simulink model "SMC_network"  (R2021a)
settings: Solver=VariableStepAuto  StartTime=0.0  StopTime=5  RelTol=1e-3
values from neighbouring files (symbols this model uses):
  C = 1e-12    [SMCCodes.m]
  eta_d = 1e27    (= 1e+27)    [SMCCodes.m]
  eta_ds = 1e5    (= 100000)    [SMCCodes.m]
  eta_q = 1e27    (= 1e+27)    [SMCCodes.m]
  eta_qs = 1e5    (= 100000)    [SMCCodes.m]
  g = -10e14    (= -1e+15)    [SMCCodes.m]
  gs = -1/Lt    (= -99.6909580301)    [SMCCodes.m]
  L = 100e-3    (= 0.1)    [SMCCodes.m]
  lambda = 1e10    (= 10000000000)    [SMCCodes.m]
  Lf = 10e-3    (= 0.01)    [SMCCodes.m]
  Lg = 0    [SMCCodes.m]
  Ll = 31e-6    (= 3.1e-05)    [SMCCodes.m]
  phi = 0.01    [SMCCodes.m]
  R = 4.33    [SMCCodes.m]
  Rf = 40e-3    (= 0.04)    [SMCCodes.m]
  RL = 0.1    [SMCCodes.m]
  Ts = 0.50e-5    (= 5e-06)    [SMCCodes.m]
undefined symbols (not defined in the file or in its folder): Ion, Lithium, sigbuilder_block
libraries: spsMeanLib x47, spsSeriesRLCBranchLib x23, simulink x22, spsFirstOrderFilterLib x10, spsIGBTDiodeLib x8, pid_lib x8, spsPWMGeneratorDCDCLib x8, spsabctodq0Lib x7, spsThreePhaseVIMeasurementLib x6, spsCurrentMeasurementLib x4, spsDiodeLib x4, spsIGBTLib x4
(part 3 of 3)

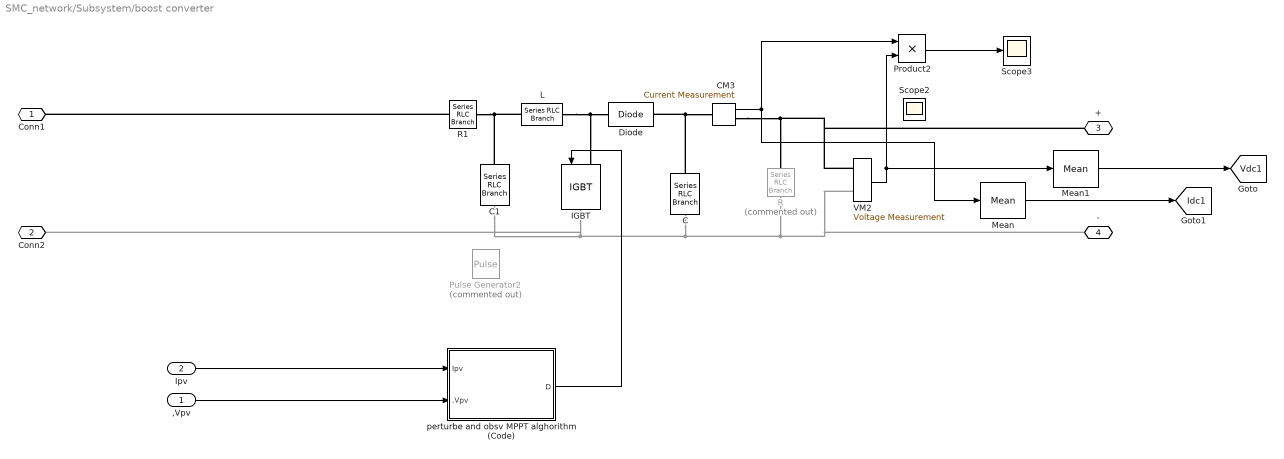
== system SMC_network/Subsystem/boost converter ==
  ,Vpv : Inport
  "Ipv " : Inport  Port=2
  C : spsSeriesRLCBranchLib/Series RLC Branch  LConnTagsString=__new0  RConnTagsString=__new0  BranchType=C  Resistance=0.01  Inductance=1.0  SetiL0=off  InitialCurrent=0  Capacitance=500e-6  Setx0=off  InitialVoltage=200  Measurements=None
  C1 : spsSeriesRLCBranchLib/Series RLC Branch  LConnTagsString=__new0  RConnTagsString=__new0  BranchType=C  Resistance=0.01  Inductance=1.0  SetiL0=off  InitialCurrent=0  Capacitance=1000e-6  Setx0=off  InitialVoltage=34.5  Measurements=None
  CM3 : spsCurrentMeasurementLib/Current Measurement  Tag=PoWeRsYsTeMmEaSuReMeNt  PhasorSimulation=off  OutputType=Magnitude  PSBequivalent=0
      settings: AttributesFormatString=\n
  Diode : spsDiodeLib/Diode  Ron=0.001  Lon=0  Vf=0.8  IC=0  UseSnubber=0  Rs=500  Cs=250e-9  Measurements=off
      settings: AttributesFormatString=\n
  IGBT : spsIGBTLib/IGBT  Ron=0.001  Lon=0  Vf=1  Tf=1e-6  Tt=2e-6  IC=0  Rs=1e5  Cs=inf  Measurements=off
  L : spsSeriesRLCBranchLib/Series RLC Branch  LConnTagsString=__new0  RConnTagsString=__new0  BranchType=L  Resistance=1.0  Inductance=168e-6  SetiL0=off  InitialCurrent=0  Capacitance=1.0  Setx0=off  InitialVoltage=0  Measurements=None
  Mean : spsMeanLib/Mean  Freq=60  Vinit=0  Ts=0
  Mean1 : spsMeanLib/Mean  Freq=60  Vinit=0  Ts=0
  Product2 : Product  RndMeth=Zero
  Pulse Generator2 : DiscretePulseGenerator  Commented=on  PulseType=Time based  Amplitude=2  Period=1/1000  PulseWidth=35
  R : spsSeriesRLCBranchLib/Series RLC Branch  Commented=on  LConnTagsString=__new0  RConnTagsString=__new0  BranchType=R  Resistance=10  Inductance=1.0  SetiL0=off  InitialCurrent=0  Capacitance=1.0  Setx0=off  InitialVoltage=0  Measurements=None
  R1 : spsSeriesRLCBranchLib/Series RLC Branch  LConnTagsString=__new0  RConnTagsString=__new0  BranchType=R  Resistance=1  Inductance=1.0  SetiL0=off  InitialCurrent=0  Capacitance=1.0  Setx0=off  InitialVoltage=0  Measurements=None
  Scope2 : Scope
  Scope3 : Scope
  VM2 : spsVoltageMeasurementLib/Voltage Measurement  Tag=PoWeRsYsTeMmEaSuReMeNt  PhasorSimulation=off  OutputType=Magnitude  PSBequivalent=0
  perturbe and obsv MPPT alghorithm (Code) : Subsystem
  Conn1 : PMIOPort  Side=Left
  Conn2 : PMIOPort  Port=2  Side=Left
  + : PMIOPort  Port=3  Side=Right
  - : PMIOPort  Port=4  Side=Right
  tag scope: Idc1=global, Vdc1=global
  wires:
  CM3/1 -> Mean/1, Product2/1
  VM2/1 -> Mean1/1, Product2/2
  perturbe and obsv MPPT alghorithm (Code)/1(D) -> IGBT/1
  Product2/1 -> Scope3/1
  "Ipv "/1 -> perturbe and obsv MPPT alghorithm (Code)/1("Ipv ")
  ,Vpv/1 -> perturbe and obsv MPPT alghorithm (Code)/2(,Vpv)
  Mean/1 -> [Idc1]
  Mean1/1 -> [Vdc1]
  connections:
  L/LConn1 -- R1/RConn1 -- C1/LConn1
  R/RConn1 -- -/RConn1 -- VM2/LConn2 -- C1/RConn1 -- Conn2/RConn1 -- IGBT/RConn1 -- C/RConn1
  L/RConn1 -- Diode/LConn1 -- IGBT/LConn1
  C/LConn1 -- CM3/LConn1 -- Diode/RConn1
  CM3/RConn1 -- R/LConn1 -- VM2/LConn1 -- +/RConn1
  R1/LConn1 -- Conn1/RConn1

== system SMC_network/Subsystem/boost converter1 ==
  ,Vpv : Inport
  "Ipv " : Inport  Port=2
  C : spsSeriesRLCBranchLib/Series RLC Branch  LConnTagsString=__new0  RConnTagsString=__new0  BranchType=C  Resistance=0.01  Inductance=1.0  SetiL0=off  InitialCurrent=0  Capacitance=500e-6  Setx0=off  InitialVoltage=200  Measurements=None
  C1 : spsSeriesRLCBranchLib/Series RLC Branch  LConnTagsString=__new0  RConnTagsString=__new0  BranchType=C  Resistance=0.01  Inductance=1.0  SetiL0=off  InitialCurrent=0  Capacitance=1000e-6  Setx0=off  InitialVoltage=34.5  Measurements=None
  CM3 : spsCurrentMeasurementLib/Current Measurement  Tag=PoWeRsYsTeMmEaSuReMeNt  PhasorSimulation=off  OutputType=Magnitude  PSBequivalent=0
      settings: AttributesFormatString=\n
  Diode : spsDiodeLib/Diode  Ron=0.00001  Lon=0  Vf=0.8  IC=0  UseSnubber=0  Rs=500  Cs=250e-9  Measurements=off
      settings: AttributesFormatString=\n
  IGBT : spsIGBTLib/IGBT  Ron=0.00001  Lon=0  Vf=1  Tf=1e-6  Tt=2e-6  IC=0  Rs=1e5  Cs=inf  Measurements=off
  L : spsSeriesRLCBranchLib/Series RLC Branch  LConnTagsString=__new0  RConnTagsString=__new0  BranchType=L  Resistance=1.0  Inductance=168e-6  SetiL0=off  InitialCurrent=0  Capacitance=1.0  Setx0=off  InitialVoltage=0  Measurements=None
  Mean : spsMeanLib/Mean  Freq=60  Vinit=0  Ts=0
  Mean1 : spsMeanLib/Mean  Freq=60  Vinit=0  Ts=0
  Product2 : Product  RndMeth=Zero
  Pulse Generator2 : DiscretePulseGenerator  Commented=on  PulseType=Time based  Amplitude=2  Period=1/1000  PulseWidth=35
  R : spsSeriesRLCBranchLib/Series RLC Branch  Commented=on  LConnTagsString=__new0  RConnTagsString=__new0  BranchType=R  Resistance=10  Inductance=1.0  SetiL0=off  InitialCurrent=0  Capacitance=1.0  Setx0=off  InitialVoltage=0  Measurements=None
  R1 : spsSeriesRLCBranchLib/Series RLC Branch  LConnTagsString=__new0  RConnTagsString=__new0  BranchType=R  Resistance=1  Inductance=1.0  SetiL0=off  InitialCurrent=0  Capacitance=1.0  Setx0=off  InitialVoltage=0  Measurements=None
  Scope2 : Scope
  Scope3 : Scope
  VM2 : spsVoltageMeasurementLib/Voltage Measurement  Tag=PoWeRsYsTeMmEaSuReMeNt  PhasorSimulation=off  OutputType=Magnitude  PSBequivalent=0
  perturbe and obsv MPPT alghorithm (Code) : Subsystem
  Conn1 : PMIOPort  Side=Left
  Conn2 : PMIOPort  Port=2  Side=Left
  + : PMIOPort  Port=3  Side=Right
  - : PMIOPort  Port=4  Side=Right
  tag scope: Idc2=global, Vdc2=global
  wires:
  ,Vpv/1 -> perturbe and obsv MPPT alghorithm (Code)/2(,Vpv)
  "Ipv "/1 -> perturbe and obsv MPPT alghorithm (Code)/1("Ipv ")
  Product2/1 -> Scope3/1
  perturbe and obsv MPPT alghorithm (Code)/1(D) -> IGBT/1
  VM2/1 -> Product2/2, Mean1/1
  CM3/1 -> Mean/1, Scope2/1, Product2/1
  Mean1/1 -> [Vdc2]
  Mean/1 -> [Idc2]
  connections:
  R1/LConn1 -- Conn1/RConn1
  +/RConn1 -- VM2/LConn1 -- R/LConn1 -- CM3/RConn1
  Diode/RConn1 -- CM3/LConn1 -- C/LConn1
  IGBT/LConn1 -- Diode/LConn1 -- L/RConn1
  C/RConn1 -- IGBT/RConn1 -- Conn2/RConn1 -- C1/RConn1 -- VM2/LConn2 -- -/RConn1 -- R/RConn1
  C1/LConn1 -- R1/RConn1 -- L/LConn1

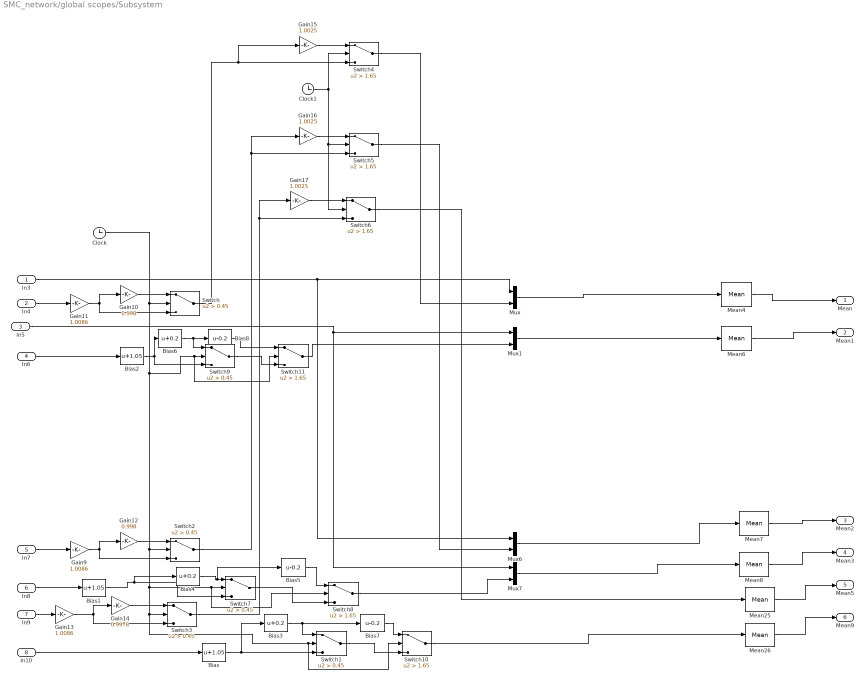
== system SMC_network/global scopes/Subsystem ==
  In3 : Inport
  In4 : Inport  Port=2
  In5 : Inport  Port=3
  In6 : Inport  Port=4
  In7 : Inport  Port=5
  In8 : Inport  Port=6
  In9 : Inport  Port=7
  In10 : Inport  Port=8
  Bias : Bias  Bias=1.05  SaturateOnIntegerOverflow=on
  Bias1 : Bias  Bias=1.05  SaturateOnIntegerOverflow=on
  Bias2 : Bias  Bias=1.05  SaturateOnIntegerOverflow=on
  Bias3 : Bias  Bias=0.2  SaturateOnIntegerOverflow=on
  Bias4 : Bias  Bias=0.2  SaturateOnIntegerOverflow=on
  Bias5 : Bias  Bias=-0.2  SaturateOnIntegerOverflow=on
  Bias6 : Bias  Bias=0.2  SaturateOnIntegerOverflow=on
  Bias7 : Bias  Bias=-0.2  SaturateOnIntegerOverflow=on
  Bias8 : Bias  Bias=-0.2  SaturateOnIntegerOverflow=on
  Clock : Clock
  Clock1 : Clock
  Gain10 : Gain  Gain=0.998
  Gain11 : Gain  Gain=1.0086
  Gain12 : Gain  Gain=0.998
  Gain13 : Gain  Gain=1.0086
  Gain14 : Gain  Gain=0.9978
  Gain15 : Gain  Gain=1.0025
  Gain16 : Gain  Gain=1.0025
  Gain17 : Gain  Gain=1.0025
  Gain9 : Gain  Gain=1.0086
  Mean{4,6..8,25..26} (6 alike) : spsMeanLib/Mean  Freq=50  Vinit=0  Ts=0
  Mux{,1,6..7} (4 alike) : Mux  Inputs=2
  Switch{,1..3,7,9} (6 alike) : Switch  Criteria=u2 > Threshold  Threshold=0.45
  Switch{4..6,8,10..11} (6 alike) : Switch  Criteria=u2 > Threshold  Threshold=1.65
  Mean : Outport
  Mean1 : Outport  Port=2
  Mean2 : Outport  Port=3
  Mean3 : Outport  Port=4
  Mean5 : Outport  Port=5
  Mean9 : Outport  Port=6
  wires:
  In3/1 -> Mux6/1, Mux/1
  In4/1 -> Gain11/1
  Clock/1 -> Switch11/2, Switch9/2, Switch2/2, Switch10/2, Switch1/2, Switch3/2, Switch8/2, Switch7/2, Switch/2
  Switch/1 -> Gain15/1, Switch4/3
  Switch2/1 -> Switch5/3, Gain16/1
  Switch3/1 -> Gain17/1, Switch6/3
  Mean4/1 -> Mean/1
  Mean8/1 -> Mean3/1
  Gain17/1 -> Switch6/1
  Gain14/1 -> Switch3/1
  Gain13/1 -> Switch3/3, Gain14/1
  Clock1/1 -> Switch4/2, Switch6/2, Switch5/2
  Gain16/1 -> Switch5/1
  In5/1 -> Mux1/1, Mux7/1
  Switch6/1 -> Mean25/1
  Mux/1 -> Mean4/1
  Mux6/1 -> Mean7/1
  Mux7/1 -> Mean8/1
  Mux1/1 -> Mean6/1
  Gain11/1 -> Switch/3, Gain10/1
  Gain15/1 -> Switch4/1
  Gain9/1 -> Gain12/1, Switch2/3
  Switch4/1 -> Mux/2
  In9/1 -> Gain13/1
  In10/1 -> Bias/1
  Mean25/1 -> Mean5/1
  Gain10/1 -> Switch/1
  Gain12/1 -> Switch2/1
  Mean26/1 -> Mean9/1
  Switch5/1 -> Mux6/2
  Mean7/1 -> Mean2/1
  Mean6/1 -> Mean1/1
  In7/1 -> Gain9/1
  In8/1 -> Bias1/1
  In6/1 -> Bias2/1
  Bias/1 -> Bias3/1, Switch1/3
  Bias3/1 -> Bias7/1, Switch1/1
  Bias1/1 -> Bias4/1, Switch7/3
  Bias4/1 -> Bias5/1, Switch7/1
  Bias5/1 -> Switch8/1
  Switch7/1 -> Switch8/3
  Bias2/1 -> Bias6/1, Switch9/3
  Bias6/1 -> Bias8/1, Switch9/1
  Switch1/1 -> Switch10/3
  Bias7/1 -> Switch10/1
  Switch10/1 -> Mean26/1
  Switch8/1 -> Mux7/2
  Switch11/1 -> Mux1/2
  Switch9/1 -> Switch11/3
  Bias8/1 -> Switch11/1

== system SMC_network/global scopes/Subsystem1 ==
  In2 : Inport
  In1 : Inport  Port=2
  Bias : Bias  Bias=-1.7  SaturateOnIntegerOverflow=on
  Bias1 : Bias  Bias=-0.58  SaturateOnIntegerOverflow=on
  Bias2 : Bias  Bias=0.5  SaturateOnIntegerOverflow=on
  Bias3 : Bias  SaturateOnIntegerOverflow=on
  Bias4 : Bias  Bias=-0.15  SaturateOnIntegerOverflow=on
  Bias5 : Bias  Bias=-0.6  SaturateOnIntegerOverflow=on
  Bias6 : Bias  Bias=-0.1  SaturateOnIntegerOverflow=on
  Bias7 : Bias  Bias=+0.1  SaturateOnIntegerOverflow=on
  Bias9 : Bias  Bias=+0.18  SaturateOnIntegerOverflow=on
  Clock : Clock
  Switch : Switch  Criteria=u2 > Threshold  Threshold=1.03
  Switch1 : Switch  Criteria=u2 > Threshold  Threshold=2.03
  Switch2 : Switch  Criteria=u2 > Threshold  Threshold=1.03
  Switch3 : Switch  Criteria=u2 > Threshold  Threshold=4.03
  Switch4 : Switch  Criteria=u2 > Threshold  Threshold=2.03
  Switch5 : Switch  Criteria=u2 > Threshold  Threshold=3.03
  Switch7 : Switch  Criteria=u2 > Threshold  Threshold=4.03
  Out1 : Outport
  Out2 : Outport  Port=2
  wires:
  In2/1 -> Bias/1
  Clock/1 -> Switch4/2, Switch7/2, Switch5/2, Switch2/2, Switch1/2, Switch3/2, Switch/2
  Bias/1 -> Bias2/1, Switch/3
  Bias2/1 -> Bias3/1, Switch/1
  Bias3/1 -> Bias5/1, Switch1/1
  Switch/1 -> Switch1/3
  Bias1/1 -> Switch2/3, Bias4/1
  Bias4/1 -> Bias6/1, Switch2/1
  Bias5/1 -> Switch3/1
  Switch1/1 -> Switch3/3
  Switch2/1 -> Switch4/3
  Bias6/1 -> Bias7/1, Switch4/1
  Switch4/1 -> Switch5/3
  Bias7/1 -> Bias9/1, Switch5/1
  Switch5/1 -> Switch7/3
  Bias9/1 -> Switch7/1
  Switch7/1 -> Out2/1
  Switch3/1 -> Out1/1
  In1/1 -> Bias1/1

== system SMC_network/global scopes/Subsystem2 ==
  In1 : Inport
  In2 : Inport  Port=2
  Bias : Bias  Bias=-0.16  SaturateOnIntegerOverflow=on
  Bias1 : Bias  Bias=-0.04  SaturateOnIntegerOverflow=on
  Bias2 : Bias  Bias=-0.03  SaturateOnIntegerOverflow=on
  Bias3 : Bias  Bias=-0.01  SaturateOnIntegerOverflow=on
  Bias4 : Bias  Bias=+0.01
  Bias5 : Bias  Bias=-0.03  SaturateOnIntegerOverflow=on
  Bias6 : Bias  Bias=+0.03  SaturateOnIntegerOverflow=on
  Bias7 : Bias  Bias=+0.03  SaturateOnIntegerOverflow=on
  Clock : Clock
  Switch : Switch  Criteria=u2 > Threshold  Threshold=1
  Switch1 : Switch  Criteria=u2 > Threshold  Threshold=2.03
  Switch2 : Switch  Criteria=u2 > Threshold  Threshold=3.03
  Switch3 : Switch  Criteria=u2 > Threshold  Threshold=1
  Switch4 : Switch  Criteria=u2 > Threshold  Threshold=4.03
  Switch5 : Switch  Criteria=u2 > Threshold  Threshold=4.03
  Out1 : Outport
  Out2 : Outport  Port=2
  wires:
  In2/1 -> Bias1/1
  In1/1 -> Bias/1
  Clock/1 -> Switch4/2, Switch2/2, Switch1/2, Switch5/2, Switch3/2, Switch/2
  Bias1/1 -> Switch/3, Bias2/1
  Bias2/1 -> Bias3/1, Switch/1
  Switch/1 -> Switch1/3
  Bias3/1 -> Bias4/1, Switch1/1
  Switch1/1 -> Switch2/3
  Bias4/1 -> Bias6/1, Switch2/1
  Bias/1 -> Bias5/1, Switch3/3
  Bias5/1 -> Bias7/1, Switch3/1
  Switch2/1 -> Switch4/3
  Bias6/1 -> Switch4/1
  Switch4/1 -> Out2/1
  Switch3/1 -> Switch5/3
  Bias7/1 -> Switch5/1
  Switch5/1 -> Out1/1

== system SMC_network/refrences/Discrete Virtual PLL ==
  note: Pierre Giroux, Gilbert Sybille
      | Power System Simulation Laboratory
      | IREQ, Hydro-Quebc
  note: Discrete Virtual PLL
  Constant4 : Constant  Value=2*pi
  Deg->Rad : Gain  Gain=pi/180  SaturateOnIntegerOverflow=on  OutDataTypeStr=Inherit: Same as input  ParamDataTypeStr=Inherit: Same as input
  Freq1 : Constant  Value=Freq
  Freq2 : Constant  Value=2*pi
  Initial Vd_Vq1 : Constant  Value=Phase
  Math Function : Math  Operator=mod  SignedPower=on  SaturateOnIntegerOverflow=on
  Mux : Mux  Inputs=2
  Product : Product  Inputs=***  InputSameDT=on  SaturateOnIntegerOverflow=on  OutDataTypeStr=Inherit: Same as first input
  Sum : Sum  InputSameDT=on  SaturateOnIntegerOverflow=on  OutDataTypeStr=Inherit: Same as first input
  Trigonometric Function : Trigonometry
  Trigonometric Function1 : Trigonometry  Operator=cos
  t : DigitalClock  SampleTime=Ts
  Freq : Outport  VectorParamsAs1DForOutWhenUnconnected=off
  Sin_Cos : Outport  Port=2  VectorParamsAs1DForOutWhenUnconnected=off
  wt : Outport  Port=3  VectorParamsAs1DForOutWhenUnconnected=off
  wires:
  Sum/1 -> Math Function/1
  t/1 -> Product/2
  Freq2/1 -> Product/3
  Freq1/1 -> Product/1, Freq/1
  Deg->Rad/1 -> Sum/2
  Initial Vd_Vq1/1 -> Deg->Rad/1
  Product/1 -> Sum/1
  Constant4/1 -> Math Function/2
  Math Function/1 -> wt/1, Trigonometric Function1/1, Trigonometric Function/1
  Trigonometric Function/1 -> Mux/1
  Trigonometric Function1/1 -> Mux/2
  Mux/1 -> Sin_Cos/1

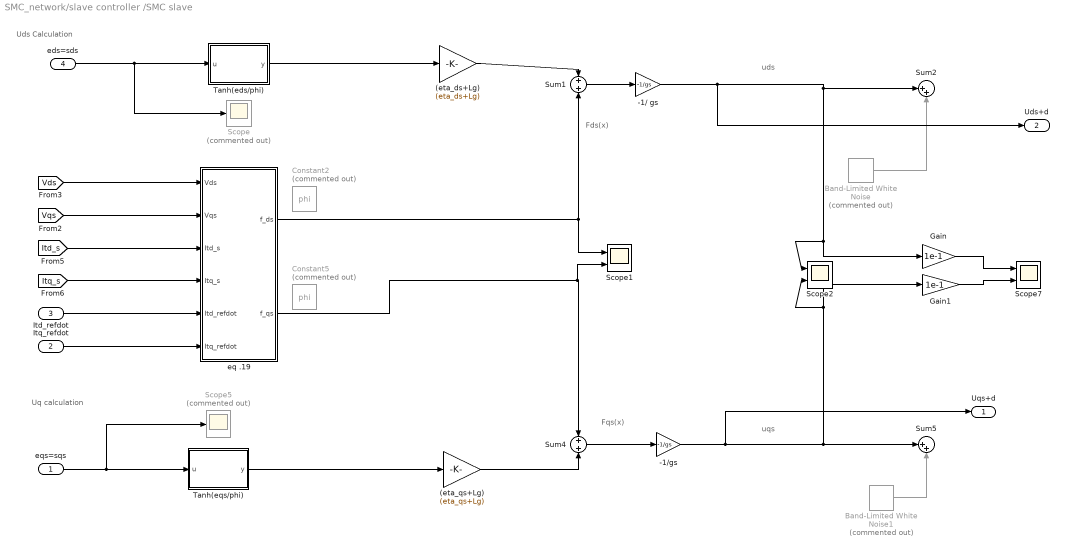
== system SMC_network/slave controller /SMC slave ==
  note: Uq calculation
  note: Uds Calculation
  note: uqs
  note: Fqs(x)
  note: Fds(x)
  note: uds
  eqs=sqs : Inport
  Itq_refdot : Inport  Port=2
  Itd_refdot : Inport  Port=3
  eds=sds : Inport  Port=4
  (eta_ds+Lg) : Gain  Gain=(eta_ds+Lg)
  (eta_qs+Lg) : Gain  Gain=(eta_qs+Lg)
  -1/ gs : Gain  Gain=-1/gs
  -1/gs : Gain  Gain=-1/gs
  Band-Limited White Noise : simulink/Sources/Band-Limited White Noise  Commented=on  Cov=[0.1]  Ts=0.002  seed=[21]
  Band-Limited White Noise1 : simulink/Sources/Band-Limited White Noise  Commented=on  Cov=[0.1]  Ts=0.002  seed=[23341]
  Constant2 : Constant  Commented=on  Value=phi
  Constant5 : Constant  Commented=on  Value=phi
  Gain : Gain  Gain=1e-1
  Gain1 : Gain  Gain=1e-1
  Scope : Scope  Commented=on
  Scope1 : Scope  NumInputPorts=2
  Scope2 : Scope  NumInputPorts=2
  Scope5 : Scope  Commented=on
  Scope7 : Scope  NumInputPorts=2
  Sum1 : Sum  Inputs=+|+
  Sum2 : Sum  Inputs=|++
  Sum4 : Sum
  Sum5 : Sum  Inputs=|++
  Tanh(eds/phi) : MATLAB Function  TreatAsAtomicUnit=on
  Tanh(eqs/phi) : MATLAB Function  TreatAsAtomicUnit=on
  eq .19 : MATLAB Function  TreatAsAtomicUnit=on
  Uqs+d : Outport
  Uds+d : Outport  Port=2
  wires:
  Tanh(eqs/phi)/1(y) -> (eta_qs+Lg)/1
  (eta_qs+Lg)/1 -> Sum4/2
  (eta_ds+Lg)/1 -> Sum1/1
  Tanh(eds/phi)/1(y) -> (eta_ds+Lg)/1
  Band-Limited White Noise1/1 -> Sum5/2
  -1/gs/1 -> Scope2/2, Gain1/1, Sum5/1, Uqs+d/1
  Sum4/1 -> -1/gs/1
  Band-Limited White Noise/1 -> Sum2/2
  -1/ gs/1 -> Uds+d/1, Gain/1, Scope2/1, Sum2/1
  Sum1/1 -> -1/ gs/1
  eds=sds/1 -> Scope/1, Tanh(eds/phi)/1(u)
  eqs=sqs/1 -> Scope5/1, Tanh(eqs/phi)/1(u)
  eq .19/1(f_ds) -> Scope1/1, Sum1/2
  eq .19/2(f_qs) -> Scope1/2, Sum4/1
  [Vds] -> eq .19/1(Vds)
  [Vqs] -> eq .19/2(Vqs)
  [Itd_s] -> eq .19/3(Itd_s)
  [Itq_s] -> eq .19/4(Itq_s)
  Itd_refdot/1 -> eq .19/5(Itd_refdot)
  Itq_refdot/1 -> eq .19/6(Itq_refdot)
  Gain/1 -> Scope7/1
  Gain1/1 -> Scope7/2

== system SMC_network/slave controller /calculation ==
  Itd_s_ref : Inport
  Itd_s : Inport  Port=2
  Discrete Derivative : simulink/Discrete/Discrete Derivative  Commented=on  gainval=1.0  ICPrevScaledInput=0.0  OutMin=[]  OutMax=[]  OutDataType=fixdt(1, 16)  OutScaling=2^-10  DoSatur=off
  First-Order Filter1 : spsFirstOrderFilterLib/First-Order Filter  FilterType=Lowpass  Tc=10e-3  Ts=0  Initialize=off  Vac_Init=[0, 0, 60]  Vdc_Init=0  PlotResponse=off  FreqRange="[0,  200,  1]"
  First-Order Filter2 : spsFirstOrderFilterLib/First-Order Filter  Commented=on  FilterType=Lowpass  Tc=20e-3  Ts=0  Initialize=off  Vac_Init=[0, 0, 60]  Vdc_Init=0  PlotResponse=off  FreqRange="[0,  200,  1]"
  Sum : Sum  Inputs=|+-
  XY Graph : simulink/Sinks/XY Graph  Commented=on  xmin=-2.5  xmax=2.5  ymin=-30  ymax=40  st=-1
  eds=sds : Outport
  tag scope: ed_s=global
  wires:
  Itd_s_ref/1 -> Sum/1
  Itd_s/1 -> Sum/2
  Sum/1 -> Discrete Derivative/1, XY Graph/1, [ed_s], eds=sds/1
  Discrete Derivative/1 -> First-Order Filter2/1
  First-Order Filter2/1 -> XY Graph/2

== system SMC_network/slave controller /calculation1 ==
  Itq_s_ref : Inport
  Itq_s : Inport  Port=2
  Discrete Derivative : simulink/Discrete/Discrete Derivative  Commented=on  gainval=1.0  ICPrevScaledInput=0.0  OutMin=[]  OutMax=[]  OutDataType=fixdt(1, 16)  OutScaling=2^-10  DoSatur=off
  First-Order Filter1 : spsFirstOrderFilterLib/First-Order Filter  Commented=on  FilterType=Lowpass  Tc=20e-3  Ts=0  Initialize=off  Vac_Init=[0, 0, 60]  Vdc_Init=0  PlotResponse=off  FreqRange="[0,  200,  1]"
  Sum : Sum  Inputs=|+-
  XY Graph : simulink/Sinks/XY Graph  Commented=on  xmin=-2.5  xmax=2.5  ymin=-20  ymax=30  st=-1
  eqs=sqs : Outport
  tag scope: eq_s=global
  wires:
  Itq_s_ref/1 -> Sum/1
  Itq_s/1 -> Sum/2
  Sum/1 -> XY Graph/1, [eq_s], eqs=sqs/1, Discrete Derivative/1
  Discrete Derivative/1 -> First-Order Filter1/1
  First-Order Filter1/1 -> XY Graph/2

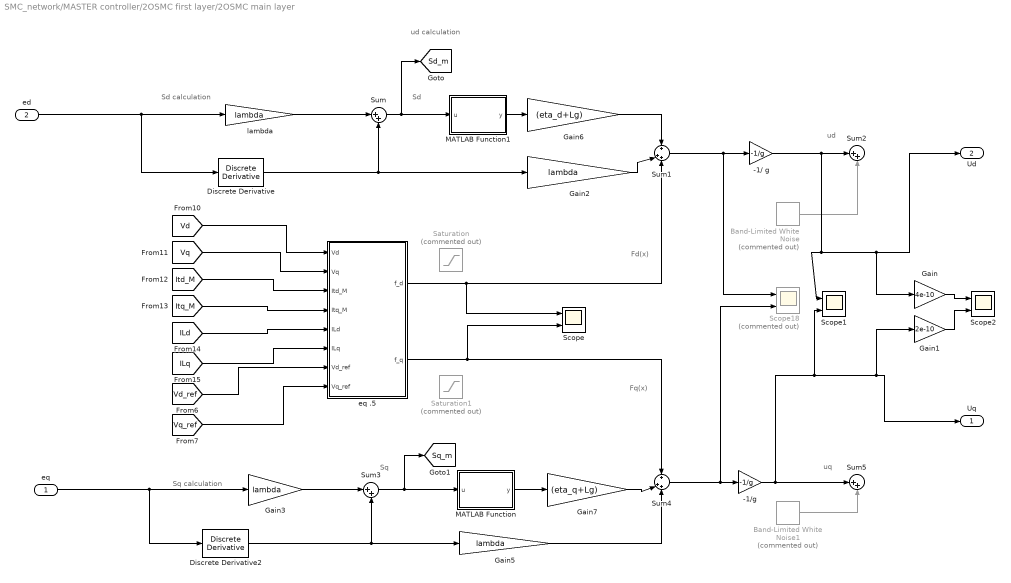
== system SMC_network/MASTER controller/2OSMC first layer/2OSMC main layer ==
  note: ud calculation
  note: ud
  note: Sq
  note: Fd(x)
  note: Sd
  note: Sd calculation
  note: Sq calculation
  note: Fq(x)
  note: uq
  eq : Inport
  ed : Inport  Port=2
  -1/ g : Gain  Gain=-1/g
  -1/g : Gain  Gain=-1/g
  Band-Limited White Noise : simulink/Sources/Band-Limited White Noise  Commented=on  Cov=[0.1]  Ts=0.002  seed=[21]
  Band-Limited White Noise1 : simulink/Sources/Band-Limited White Noise  Commented=on  Cov=[0.1]  Ts=0.002  seed=[23341]
  Discrete Derivative : simulink/Discrete/Discrete Derivative  gainval=1.0  ICPrevScaledInput=0.0  OutMin=[]  OutMax=[]  OutDataType=fixdt(1, 16)  OutScaling=2^-10  DoSatur=off
  Discrete Derivative2 : simulink/Discrete/Discrete Derivative  gainval=1.0  ICPrevScaledInput=0.0  OutMin=[]  OutMax=[]  OutDataType=fixdt(1, 16)  OutScaling=2^-10  DoSatur=off
  Gain : Gain  Gain=4e-10
  Gain1 : Gain  Gain=2e-10
  Gain2 : Gain  Gain=lambda
  Gain3 : Gain  Gain=lambda
  Gain5 : Gain  Gain=lambda
  Gain6 : Gain  Gain=(eta_d+Lg)
  Gain7 : Gain  Gain=(eta_q+Lg)
  MATLAB Function : MATLAB Function  TreatAsAtomicUnit=on
  MATLAB Function1 : MATLAB Function  TreatAsAtomicUnit=on
  Saturation : Saturate  Commented=on  UpperLimit=65e22  LowerLimit=0
  Saturation1 : Saturate  Commented=on  UpperLimit=110e12  LowerLimit=0
  Scope : Scope  NumInputPorts=2
  Scope1 : Scope  NumInputPorts=2
  Scope18 : Scope  Commented=on  NumInputPorts=2
  Scope2 : Scope  NumInputPorts=2
  Sum{,2..3,5} (4 alike) : Sum  Inputs=|++
  Sum1 : Sum  Inputs=+|++
  Sum4 : Sum  Inputs=+|++
  eq .5 : MATLAB Function  TreatAsAtomicUnit=on
  lambda : Gain  Gain=lambda
  Uq : Outport
  Ud : Outport  Port=2
  tag scope: Sd_m=global, Sq_m=global
  wires:
  ed/1 -> Discrete Derivative/1, lambda/1
  Gain2/1 -> Sum1/2
  Sum/1 -> [Sd_m], MATLAB Function1/1(u)
  Sum1/1 -> Scope18/1, -1/ g/1
  Band-Limited White Noise/1 -> Sum2/2
  Sum4/1 -> -1/g/1, Scope18/2
  Sum3/1 -> [Sq_m], MATLAB Function/1(u)
  Band-Limited White Noise1/1 -> Sum5/2
  MATLAB Function1/1(y) -> Gain6/1
  Gain6/1 -> Sum1/1
  Gain7/1 -> Sum4/2
  MATLAB Function/1(y) -> Gain7/1
  Gain5/1 -> Sum4/3
  eq/1 -> Discrete Derivative2/1, Gain3/1
  -1/g/1 -> Scope1/2, Gain1/1, Uq/1, Sum5/1
  -1/ g/1 -> Scope1/1, Ud/1, Gain/1, Sum2/1
  eq .5/2(f_q) -> Scope/2, Sum4/1
  eq .5/1(f_d) -> Sum1/3, Scope/1
  [Vd] -> eq .5/1(Vd)
  [Vq] -> eq .5/2(Vq)
  [Itd_M] -> eq .5/3(Itd_M)
  [Itq_M] -> eq .5/4(Itq_M)
  [ILd] -> eq .5/5(ILd)
  [ILq] -> eq .5/6(ILq)
  Discrete Derivative/1 -> Sum/2, Gain2/1
  lambda/1 -> Sum/1
  Gain3/1 -> Sum3/1
  Discrete Derivative2/1 -> Sum3/2, Gain5/1
  [Vd_ref] -> eq .5/7(Vd_ref)
  [Vq_ref] -> eq .5/8(Vq_ref)
  Gain1/1 -> Scope2/2
  Gain/1 -> Scope2/1

== system SMC_network/MASTER controller/2OSMC first layer/calculation ==
  Vd : Inport
  Vd_ref : Inport  Port=2
  Discrete Derivative : simulink/Discrete/Discrete Derivative  Commented=on  gainval=1.0  ICPrevScaledInput=0.0  OutMin=[]  OutMax=[]  OutDataType=fixdt(1, 16)  OutScaling=2^-10  DoSatur=off
  First-Order Filter : spsFirstOrderFilterLib/First-Order Filter  Commented=on  FilterType=Lowpass  Tc=20e-3  Ts=0  Initialize=off  Vac_Init=[0, 0, 60]  Vdc_Init=0  PlotResponse=off  FreqRange="[0,  200,  1]"
  Sum : Sum  Inputs=+-
  XY Graph : simulink/Sinks/XY Graph  Commented=on  xmin=-25  xmax=25  ymin=-300  ymax=300  st=-1
  ed : Outport
  tag scope: ed=global
  wires:
  Sum/1 -> XY Graph/1, [ed], ed/1, Discrete Derivative/1
  Vd_ref/1 -> Sum/1
  Vd/1 -> Sum/2
  First-Order Filter/1 -> XY Graph/2
  Discrete Derivative/1 -> First-Order Filter/1

== system SMC_network/MASTER controller/2OSMC first layer/calculation1 ==
  Vq : Inport
  Vq_ref : Inport  Port=2
  Discrete Derivative : simulink/Discrete/Discrete Derivative  Commented=on  gainval=1.0  ICPrevScaledInput=0.0  OutMin=[]  OutMax=[]  OutDataType=fixdt(1, 16)  OutScaling=2^-10  DoSatur=off
  First-Order Filter : spsFirstOrderFilterLib/First-Order Filter  Commented=on  FilterType=Lowpass  Tc=20e-3  Ts=0  Initialize=off  Vac_Init=[0, 0, 60]  Vdc_Init=0  PlotResponse=off  FreqRange="[0,  200,  1]"
  Sum : Sum  Inputs=+-  AccumDataTypeStr=double
  XY Graph : simulink/Sinks/XY Graph  Commented=on  xmin=-10  xmax=10  ymin=-200  ymax=200  st=-1
  eq : Outport
  tag scope: eq=global
  wires:
  Vq_ref/1 -> Sum/1
  Vq/1 -> Sum/2
  Sum/1 -> Discrete Derivative/1, XY Graph/1, [eq], eq/1
  Discrete Derivative/1 -> First-Order Filter/1
  First-Order Filter/1 -> XY Graph/2

== system SMC_network/Subsystem/boost converter/perturbe and obsv MPPT alghorithm (Code) ==
  "Ipv " : Inport
  ,Vpv : Inport  Port=2
  MATLAB Function : MATLAB Function  TreatAsAtomicUnit=on
  Saturation1 : Saturate  LowerLimit=0  ZeroCross=off
  duty cyle : Subsystem
  D : Outport
  wires:
  Saturation1/1 -> duty cyle/1(In1)
  MATLAB Function/1(D) -> Saturation1/1
  duty cyle/1("duty ") -> D/1
  "Ipv "/1 -> MATLAB Function/1(Ipv)
  ,Vpv/1 -> MATLAB Function/2(Vpv)

== system SMC_network/Subsystem/boost converter1/perturbe and obsv MPPT alghorithm (Code) ==
  "Ipv " : Inport
  ,Vpv : Inport  Port=2
  MATLAB Function : MATLAB Function  TreatAsAtomicUnit=on
  Saturation1 : Saturate  LowerLimit=0  ZeroCross=off
  duty cyle : Subsystem
  D : Outport
  wires:
  ,Vpv/1 -> MATLAB Function/2(Vpv)
  "Ipv "/1 -> MATLAB Function/1(Ipv)
  duty cyle/1("duty ") -> D/1
  MATLAB Function/1(D) -> Saturation1/1
  Saturation1/1 -> duty cyle/1(In1)

== system SMC_network/Subsystem/boost converter/perturbe and obsv MPPT alghorithm (Code)/duty cyle ==
  In1 : Inport
  Compare To Zero : simulink/Logic and Bit Operations/Compare To Zero  relop=>=  OutDataTypeStr=boolean
  Repeating Sequence : simulink/Sources/Repeating Sequence  rep_seq_t=[0 1e-6]  rep_seq_y=[0 1]
  Subtract : Sum  Inputs=+-
  "duty " : Outport
  wires:
  Repeating Sequence/1 -> Subtract/2
  In1/1 -> Subtract/1
  Subtract/1 -> Compare To Zero/1
  Compare To Zero/1 -> "duty "/1

== system SMC_network/Subsystem/boost converter1/perturbe and obsv MPPT alghorithm (Code)/duty cyle ==
  In1 : Inport
  Compare To Zero : simulink/Logic and Bit Operations/Compare To Zero  relop=>=  OutDataTypeStr=boolean
  Repeating Sequence : simulink/Sources/Repeating Sequence  rep_seq_t=[0 1e-6]  rep_seq_y=[0 1]
  Subtract : Sum  Inputs=+-
  "duty " : Outport
  wires:
  Compare To Zero/1 -> "duty "/1
  Subtract/1 -> Compare To Zero/1
  In1/1 -> Subtract/1
  Repeating Sequence/1 -> Subtract/2

== matlab function SMC_network/MASTER controller/2OSMC first layer/2OSMC main layer/eq .5 ==
  settings: sampleTime=Ts
  data: Vd input; f_d output size=[1 1]; Vq input; Itd_M input; Itq_M input; ILd input; ILq input; f_q output size=[1 1]; Vd_ref input; Vq_ref input
function [f_d,f_q]= fcn(Vd,Vq,Itd_M,Itq_M,ILd,ILq,Vd_ref,Vq_ref)
omega0= 314 ; 
Lf = 10e-3;
Rf=  40e-3;
RL=0.1;%transmission
Ll= 31e-6;%transmission
R=4.33;
L= 100e-3;
C= 1e-12;
Rl = 0.1;%load inductive branch resistanse
% Vd_ref=311;
% Vq_ref= 0;
Rt= Rf +RL;
Lt = Lf + Ll;
% g= -1/(Lt*C);
f_d=((omega0^2) - (1/(R*C)^2) + (1/(Lt*C)) + (1/(L*C)))*Vd + ((2*omega0)/(R*C))*Vq + ((1/(R*C^2)) + (Rt/(Lt*C)))*Itd_M - ((2*omega0)/C)*Itq_M - ((1/(R*C^2)) + (Rl/(L*C)))*ILd + ((2*omega0)/C)*ILq +(-1/(Lt*C))*Vd_ref ;
f_q = -((2*omega0)/(R*C))*Vd + ((omega0^2) - (1/(R*C)^2) + (1/(Lt*C)) + (1/(L*C)))*Vq + ((2*omega0)/C)*Itd_M +((1/(R*C^2)) +(Rt/(Lt*C)))*Itq_M - ((2*omega0)/C)*ILd - ((1/(R*C^2)) + (Rl/(L*C)))*ILq+ (-1/(Lt*C))*Vq_ref;
% f_dmax=65e22;%upper bound
% f_qmax=110e12;%upper bound

== matlab function SMC_network/slave controller /SMC slave/Tanh(eds//phi) ==
  data: u input; y output
function y = fcn(u)
phi=0.01;
y = tanh(u/phi);

== matlab function SMC_network/slave controller /SMC slave/Tanh(eqs//phi) ==
  data: u input; y output
function y = fcn(u)
phi=0.01;
y = tanh(u/phi);

== matlab function SMC_network/slave controller /SMC slave/eq .19 ==
  data: Vds input; Vqs input; Itd_s input; Itq_s input; Itd_refdot input; Itq_refdot input; f_ds output size=[1 1] [..32e4]; f_qs output size=[1 1] [..11e4]
function [f_ds,f_qs]= fcn(Vds,Vqs,Itd_s,Itq_s,Itd_refdot,Itq_refdot)
omega0= 314;
Rf=  40e-3;%filter resistance
Lf = 10e-3;%filter inductance
RL=0.1;%%Transmission line resistance
Ll= 31e-6;%%Transmission line inductance

Rt= Rf +RL;
Lt = Lf + Ll;
%  gs= -1/Lt;
% f_dsmax=32e4;
% f_qsmax=11e4;

f_ds = (1/Lt)*Vds + (Rt/Lt)*Itd_s - (omega0)*Itq_s + Itd_refdot;
f_qs = (1/Lt)*Vqs + (omega0)*Itd_s + (Rt/Lt)*Itq_s + Itq_refdot;
% if abs(f_ds)<=f_dsmax
%     f_ds = (1/Lt)*Vds + (Rt/Lt)*Itd_s - (omega0)*Itq_s + Itd_refdot;
% end

% if abs(f_qs)<=f_qsmax
%     f_qs = (1/Lt)*Vqs + omega0*Itd_s + (Rt/Lt)*Itq_s + Itq_refdot;
% end

== matlab function SMC_network/Subsystem3/MATLAB Function1 ==
  data: Itq_s input; Q_S output; Vds input
function Q_S = fcn(Itq_s,Vds)

Q_S =-3/2*(Vds*Itq_s);

== matlab function SMC_network/DG unit 1/MPPT PnO/MATLAB Function ==
  settings: updateMethod=DISCRETE  sampleTime=1e-4
  data: Vpv input; D output; Ipv input
function D = PandO(Vpv,Ipv)

persistent Dold Pold Vold


if isempty(Dold)
    Dold = 0.35;
    Vold = 29.5;
    Pold = 252.81;
end


deltaD = 0.001;

Ppv = Vpv*Ipv;

if (Ppv-Pold) ~= 0
    if (Ppv-Pold) > 0
        if (Vpv-Vold) > 0
            D = Dold - deltaD;
        else
            D = Dold + deltaD;
        end
    else
        if (Vpv-Vold) > 0
            D = Dold + deltaD;
        else
            D = Dold - deltaD;
        end        
    end
else
    D = Dold;
end

Dold = D;
Vold = Vpv;
Pold = Ppv;

== matlab function SMC_network/DG UNIT 2/MPPT PnO/MATLAB Function ==
  settings: updateMethod=DISCRETE  sampleTime=1e-4
  data: Vpv input; D output; Ipv input
function D = PandO(Vpv,Ipv)

persistent Dold Pold Vold


if isempty(Dold)
    Dold = 0.35;
    Vold = 17;
    Pold = 120;
end


deltaD = 0.001;

Ppv = Vpv*Ipv;

if (Ppv-Pold) ~= 0
    if (Ppv-Pold) > 0
        if (Vpv-Vold) > 0
            D = Dold - deltaD;
        else
            D = Dold + deltaD;
        end
    else
        if (Vpv-Vold) > 0
            D = Dold + deltaD;
        else
            D = Dold - deltaD;
        end        
    end
else
    D = Dold;
end

Dold = D;
Vold = Vpv;
Pold = Ppv;

== matlab function SMC_network/Subsystem/boost converter/perturbe and obsv MPPT alghorithm (Code)/MATLAB Function ==
  settings: updateMethod=DISCRETE
  data: Ipv input; D output; Vpv input
function D = PandO(Ipv ,Vpv)

persistent Dpref Ppref Vpref

if isempty(Dpref)
    Dpref= 1;
    Vpref = 23;
    Ppref = 169.9;
end
deltaD = 150e-5;
Ppv=Vpv*Ipv;

if (Ppv-Ppref) ~= 0
    if (Ppv-Ppref) > 0
        if (Vpv-Vpref) > 0
            D = Dpref - deltaD;
        else
            D=Dpref + deltaD;
        end
    else
        if (Vpv-Vpref) > 0
            D=Dpref + deltaD ;
        else
            D=Dpref - deltaD ;
        end
    end
else
    D= Dpref;
end

%update 
Dpref=D;
Vpref=Vpv;
Ppref= Ppv;

== matlab function SMC_network/Subsystem/boost converter1/perturbe and obsv MPPT alghorithm (Code)/MATLAB Function ==
  settings: updateMethod=DISCRETE
  data: Ipv input; D output; Vpv input
function D = PandO(Ipv ,Vpv)

persistent Dpref Ppref Vpref

if isempty(Dpref)
    Dpref= 1;
    Vpref = 23;
    Ppref = 169.9;
end
deltaD = 150e-5;
Ppv=Vpv*Ipv;

if (Ppv-Ppref) ~= 0
    if (Ppv-Ppref) > 0
        if (Vpv-Vpref) > 0
            D = Dpref - deltaD;
        else
            D=Dpref + deltaD;
        end
    else
        if (Vpv-Vpref) > 0
            D=Dpref + deltaD ;
        else
            D=Dpref - deltaD ;
        end
    end
else
    D= Dpref;
end

%update 
Dpref=D;
Vpref=Vpv;
Ppref= Ppv;

== matlab function SMC_network/Subsystem1/MATLAB Function ==
  data: ILd input; pL output; Vd input
function pL = fcn(ILd,Vd)

pL =3/2*(Vd*ILd);

== matlab function SMC_network/Subsystem1/MATLAB Function1 ==
  data: ILq input; QL output; Vd input
function QL = fcn(ILq,Vd)

QL =-3/2*(Vd*ILq);

== matlab function SMC_network/Subsystem2/MATLAB Function ==
  data: Itd_M input; p_M output; Vd input
function p_M = fcn(Itd_M,Vd)

p_M =3/2*(Vd*Itd_M);

== matlab function SMC_network/Subsystem2/MATLAB Function1 ==
  data: Itq_M input; Q_M output; Vd input
function Q_M = fcn(Itq_M,Vd)

Q_M =-3/2*(Vd*Itq_M);

== matlab function SMC_network/Subsystem3/MATLAB Function ==
  data: Itd_s input; p_S output; Vds input
function p_S = fcn(Itd_s,Vds)

p_S =3/2*(Vds*Itd_s);

== matlab function SMC_network/MASTER controller/2OSMC first layer/2OSMC main layer/MATLAB Function ==
  data: u input; y output
function y = fcn(u)
phi=0.01;
y = tanh(u/phi);

== matlab function SMC_network/POWER SHARING/power sharing1 ==
  data: Vir_star_d output; Itd_M input; Itd_s input
function Vir_star_d  = fcn(Itd_M,Itd_s)


 Vir_star_d = 1.33*(Itd_M + Itd_s )/2 ;

== matlab function SMC_network/POWER SHARING/power sharing2 ==
  data: Vir_star_q output; Itq_M input; Itq_s input
function Vir_star_q  = fcn(Itq_M,Itq_s)


 Vir_star_q = 1.33*(Itq_M + Itq_s)/2 ;

== matlab function SMC_network/MASTER controller/2OSMC first layer/2OSMC main layer/MATLAB Function1 ==
  data: u input; y output
function y = fcn(u)
phi=0.01;
y = tanh(u/phi);
